simulink model "Copy_of_dop"  (R2023b)
settings: Solver=ode3  StartTime=0.0  StopTime=5  FixedStep=0.001  RelTol=1e-3
libraries: cstblocks x1
settings Model: Creator=PC  LastModifiedBy=ASUS
settings DebuggingCC: UnconnectedInputMsg=warning  UnconnectedOutputMsg=warning  UnconnectedLineMsg=warning
settings ModelReferenceCC: EnableRefExpFcnMdlSchedulingChecks=on
settings RTWCC: DLArmComputeVersion=19.05

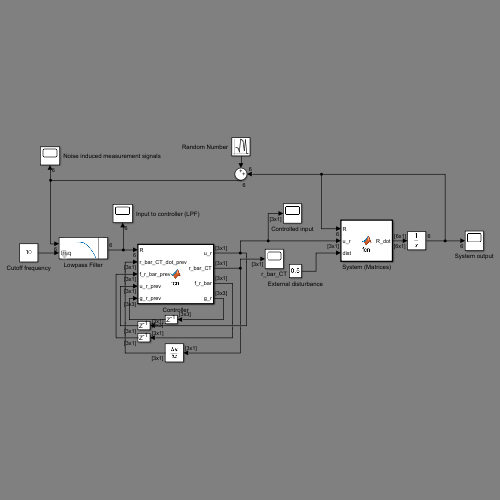
[thumbnail: Simulink's stored preview of the top-level diagram]
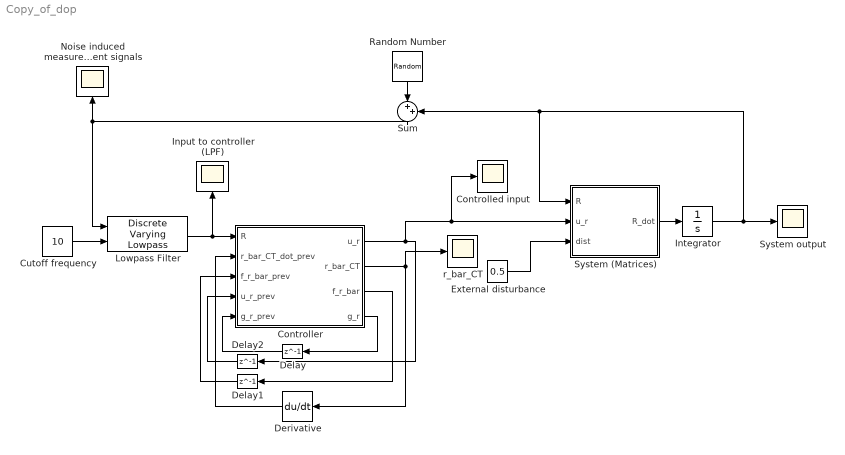
== system Copy_of_dop ==
  Controlled input : Scope
  Controller : MATLAB Function  TreatAsAtomicUnit=on
  Cutoff frequency : Constant  Value=10  SampleTime=0.001
  Delay : Delay  DelayLength=1  InitialCondition=0
  Delay1 : Delay  DelayLength=1  InitialCondition=0
  Delay2 : Delay  DelayLength=1  InitialCondition=0
  Derivative : Derivative
  External disturbance : Constant  Value=0.5  SampleTime=0.001
  Input to controller (LPF) : Scope
  Integrator : Integrator  InitialCondition=[0;-2; 0; 0; 0; 0]
  Lowpass Filter : cstblocks/Linear Parameter Varying/Discrete Varying Lowpass  N=1  w0=0  Ts=0.01
  Noise induced measurement signals : Scope
  Random Number : RandomNumber  Variance=0.001  SampleTime=0.001
  Sum : Sum  Inputs=|++
  System (Matrices) : MATLAB Function  TreatAsAtomicUnit=on
  System output : Scope
  r_bar_CT : Scope
  wires:
  Controller/1(u_r) -> Controlled input/1, System (Matrices)/2(u_r), Delay2/1
  System (Matrices)/1(R_dot) -> Integrator/1
  Controller/2(r_bar_CT) -> Derivative/1, r_bar_CT/1
  Integrator/1 -> System output/1, Sum/2, System (Matrices)/1(R)
  Cutoff frequency/1 -> Lowpass Filter/2
  Lowpass Filter/1 -> Controller/1(R), Input to controller (LPF)/1
  Sum/1 -> Lowpass Filter/1, Noise induced measurement signals/1
  Random Number/1 -> Sum/1
  External disturbance/1 -> System (Matrices)/3(dist)
  Controller/4(g_r) -> Delay/1
  Controller/3(f_r_bar) -> Delay1/1
  Derivative/1 -> Controller/2(r_bar_CT_dot_prev)
  Delay/1 -> Controller/5(g_r_prev)
  Delay1/1 -> Controller/3(f_r_bar_prev)
  Delay2/1 -> Controller/4(u_r_prev)

== matlab function Copy_of_dop/Controller ==
  data: R input; u_r output; r_bar_CT output; r_bar_CT_dot_prev input; f_r_bar_prev input; u_r_prev input; g_r_prev input; f_r_bar output; g_r output
function [u_r,r_bar_CT, f_r_bar, g_r] = fcn(R, r_bar_CT_dot_prev, f_r_bar_prev,u_r_prev, g_r_prev)
G=6.673*(10.^(-11));
M=6*10^24;
rad=500000;
w = sqrt(G*M/(rad^3));
x_CT = R(1);
y_CT = R(2);
z_CT = R(3);
x_CT_dot = R(4);
y_CT_dot = R(5);
z_CT_dot = R(6);
kx = 2;
ky = 2;                                % Kx, Ky, Kz=0 is a bad idea, it doesn't even control
kz = 2;                                %increasing Kx, Ky, Kz increases peak overshoot
K = 10*eye(3);                         %what is K and Kx,y,z doing? what is the difference?
x_bar_CT = x_CT_dot + kx*x_CT;
y_bar_CT = y_CT_dot + ky*y_CT;
z_bar_CT = z_CT_dot + kz*z_CT;
f_r_bar = [(kx*x_CT_dot) + (2*w*y_CT_dot) + (3*(w.^2)*x_CT);(ky*y_CT_dot) - (2*w*x_CT_dot);(kz*z_CT_dot) - ((w.^2)*z_CT)]; %f_r_bar = f_r + k*r_CT_dot
g_r = 2*eye(3);                        %decreasing the constant increases oscillations, increasing the same decreases the oscillations
r_bar_CT = [x_bar_CT;y_bar_CT;z_bar_CT]; 

f_d = r_bar_CT_dot_prev-f_r_bar_prev-g_r_prev*u_r_prev;


u_r = inv(g_r)*(-f_r_bar - K*r_bar_CT );

== matlab function Copy_of_dop/System (Matrices) ==
  data: R input; u_r input; R_dot output; dist input
function R_dot  = fcn(R,u_r,dist)
G=6.673*(10.^(-11));
M=6*10^24;
rad=500000;
w = sqrt(G*M/(rad^3));
A=[0 0 0 1 0 0; 0 0 0 0 1 0; 0 0 0 0 0 1; 3*w*w 0 0 0 2*w 0; 0 0 0 -2*w 0 0;0 0 -w*w 0 0 0];
B=[0 0 0;0 0 0;0 0 0;2 0 0; 0 2 0; 0 0 2];
R_dot = A*R + B*u_r + dist.*[0;0;0;1;1;1];
